simulink model "SinglePhaseFullWaveFourDiodes"  (R2020a)
settings: Solver=VariableStepAuto  StartTime=0.0  StopTime=0.033  RelTol=1e-3
libraries: powerlib x10
settings Model: Creator=Naeem Mohammad  LastModifiedBy=Naeem Mohammad

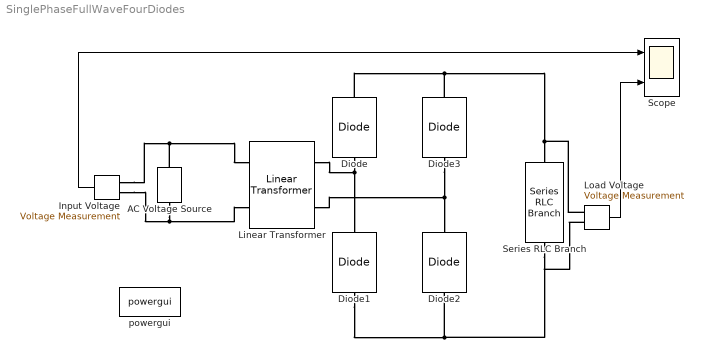
== system SinglePhaseFullWaveFourDiodes ==
  " Input Voltage" : powerlib/Measurements/Voltage Measurement  PhasorSimulation=off  OutputType=Complex  PSBequivalent=0
  AC Voltage Source : powerlib/Electrical Sources/AC Voltage Source  Amplitude=110  Phase=0  Frequency=60  SampleTime=0  Measurements=None  BusType=swing  Pref=10e3  Qref=0  Qmin=-inf  Qmax=+inf
  Diode{,1..3} (4 alike) : powerlib/Power Electronics/Diode  Ron=0.001  Lon=0  Vf=0.8  IC=0  UseSnubber=0  Rs=500  Cs=250e-9  Measurements=off
  Linear Transformer : powerlib/Elements/Linear Transformer  UNITS=pu  NominalPower=[ 40 60 ]  winding1="[ 110  0.002  0.08 ]"  winding2="[ 12  0.002  0.08 ]"  ThreeWindings=off  winding3=[ 315e3 0.002 0.08 ]  RmLm=[ 500 500 ]  Measurements=None  DataType=off
  Load Voltage : powerlib/Measurements/Voltage Measurement  PhasorSimulation=off  OutputType=Complex  PSBequivalent=0
  Scope : Scope  NumInputPorts=2
  Series RLC Branch : powerlib/Elements/Series RLC Branch  LConnTagsString=__new0  RConnTagsString=__new0  BranchType=R  Resistance=10  Inductance=1e-3  SetiL0=off  InitialCurrent=0  Capacitance=1e-6  Setx0=off  InitialVoltage=0  Measurements=None
  powergui : powerlib/powergui  Priority=1  SimulationMode=Continuous  SampleTime=50e-6  frequency=60  Iterations=50  frequencyindice=60  Pbase=100e6  ErrMax=1e-4  UnitsV=kV  UnitsW=MW  buscounter=0  FunctionMessages=off  echomessages=off  EnableUseOfTLC=off  CurrentSourceSwitches=off  DisableSnubberDevices=off  DisableRonSwitches=off  DisableVfSwitches=off  DisplayEquations=off  AutomaticDiscreteSolvers=off  SolverType=Tustin/Backward Euler (TBE)  Interpol=off  ExternalGateDelay=off  methode=off  Ts=100  x0status=blocks  SPID=on  SwTol=0  HookPort=off  NonlinearTolerance=1e-4  nMaxIteration=100  ContinueOnMaxIteration=off  RestoreLinks=warning  ResistiveCurrentMeasurement=off  Frange=[0:2:500]  Ylog=off  Xlog=on  ShowGrid=off  save=off  variable=ZData  structure=0  ZoomFFT=off  StartTime=0.0  cycles=1  DisplayStyle=1  fundamental=60  FreqAxis=off  MaxFrequency=1000  frequencyindicesteady=1  RmsSteady=1  display=off
  wires:
  " Input Voltage"/1 -> Scope/1
  Load Voltage/1 -> Scope/2
  connections:
  AC Voltage Source/RConn1 -- " Input Voltage"/LConn1 -- Linear Transformer/LConn1
  " Input Voltage"/LConn2 -- AC Voltage Source/LConn1 -- Linear Transformer/LConn2
  Diode/LConn1 -- Linear Transformer/RConn1 -- Diode1/RConn1
  Diode3/LConn1 -- Diode2/RConn1 -- Linear Transformer/RConn2
  Diode/RConn1 -- Diode3/RConn1 -- Load Voltage/LConn1 -- Series RLC Branch/LConn1
  Diode1/LConn1 -- Load Voltage/LConn2 -- Series RLC Branch/RConn1 -- Diode2/LConn1
